simulink model "subsystemExample"  (R2015a)
settings: Solver=ode45  StartTime=0.0  StopTime=10.0  RelTol=1e-3
settings Model: Creator=John  LastModifiedBy=John

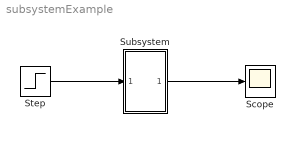
== system subsystemExample ==
  Scope : Scope
  Step : Step  SampleTime=0
  Subsystem : Subsystem
  wires:
  Step/1 -> Subsystem/1(In1)
  Subsystem/1(Out1) -> Scope/1

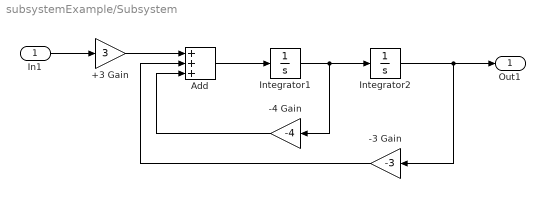
== system subsystemExample/Subsystem ==
  In1 : Inport
  +3 Gain : Gain  Gain=3
  -3 Gain : Gain  Gain=-3
  -4 Gain : Gain  Gain=-4
  Add : Sum  Inputs=+++
  Integrator1 : Integrator
  Integrator2 : Integrator  InitialCondition=0.5
  Out1 : Outport
  wires:
  Integrator1/1 -> -4 Gain/1, Integrator2/1
  -3 Gain/1 -> Add/2
  Integrator2/1 -> Out1/1, -3 Gain/1
  -4 Gain/1 -> Add/3
  Add/1 -> Integrator1/1
  In1/1 -> +3 Gain/1
  +3 Gain/1 -> Add/1
